simulink model "UNIFIER_dyn1"  (R2023b)
settings: Solver=VariableStepAuto  StartTime=0.0  StopTime=t_sim  RelTol=1e-3
InitFcn:
  | UNIFIER_LOAD
values from neighbouring files (symbols this model uses):
  b = 20.11467    [UNIFIER_LOAD.mat]
  c = 1.43676    [UNIFIER_LOAD.mat]
  dp_DEP =     [UNIFIER_LOAD.mat]
  dp_FUSE_FIN =     [UNIFIER_LOAD.mat]
  dp_HTU =     [UNIFIER_LOAD.mat]
  dp_VTAIL =     [UNIFIER_LOAD.mat]
  dp_VTAIL_INDUCED =     [UNIFIER_LOAD.mat]
  dp_WING_root =     [UNIFIER_LOAD.mat]
  dp_WING_tip =     [UNIFIER_LOAD.mat]
  I = [23600  0  -1740; 0  89800  0; -1740  0  102000]    [UNIFIER_LOAD.mat]
  m = 7057    [UNIFIER_LOAD.mat]
  rho0 = 1.11164259067    [UNIFIER_LOAD.mat]
  S = 29.98388    [UNIFIER_LOAD.mat]
  u0 = [0 0 0 0.436332312999 1 0 0]    [UNIFIER_LOAD.mat]    (also in UNIFIER_ROMdyn_w.m = X0(3); UNIFIER_dynamics.m = u; UNIFIER_dynamics0.m = u; UNIFIER_forces.m = u)
  Vrw0 = [18.7938524157 0 6.84040286651]    [UNIFIER_LOAD.mat]    (also in UNIFIER_dynamics.m = x(4:6); UNIFIER_dynamics0.m = x(4:6); UNIFIER_forces.m = x(4:6); UNIFIER_forces0.m = x(4:6))
  vtail_nodes = [-16.4894695282 -2.83441376686 -2.73765826225 -16.1370849609 -2.45649194717 -2.44886755943 -15.8320636749 -2.07857012749 -2.1468129158 -15.5873622894 -1.7006483078 -1.90353524685 ... (48 elements, 3x16)]    [UNIFIER_LOAD.mat]
  wing_nodes = [-7.70795631409 -9.67500019073 -0.98178178072 -7.66801691055 -8.6313495636 -1.01726543903 -7.65512371063 -7.83034992218 -1.03603482246 -7.6036362648 -6.84600019455 -1.09595656395 ... (42 elements, 3x14)]    [UNIFIER_LOAD.mat]
  x0 = [0 0 -1000 18.7938524157 0 6.84040286651 0 0.349065850399 0 0 0 0]    [UNIFIER_LOAD.mat]    (also in UNIFIER_ROMdyn_w.m = X0(1); UNIFIER_dynamics.m = x; UNIFIER_dynamics0.m = x; UNIFIER_forces.m = x)
  xyz_cg = [-8.09 0 -0.2]    [UNIFIER_LOAD.mat]
  xyz_DEP = [-6.9629998 -10.05 -0.90899998 -6.921 -8.4499998 -0.792 -6.8660002 -6.8499999 -0.82300001 -6.8099999 -5.25 -0.85000002 ... (36 elements, 3x12)]    [UNIFIER_LOAD.mat]
undefined symbols (not defined in the file or in its folder): OBM, unifier_obm
libraries: sharedutil x7, aerolibtransform2 x4, sharedtransform x2, matrix_library x1, shared6dofsys x1, shared6dof x1, simulink x1
(part 3 of 3)

== system UNIFIER_dyn1/UNIFIER OBM/Aero/WingForces/Right/WingRootForces/WingRootPreLookup ==
  flap_defl : Inport
  alpha : Inport  Port=2
  V_node : Inport  Port=3
  DEP_J : Inport  Port=4
  Constant8 : Constant  Value=0:4
  Prelookup : PreLookup  BreakpointsData=dp_WING_root.flap_defl  IndexSearchMethod=Linear search  BeginIndexSearchUsingPreviousIndexResult=on  UseLastBreakpoint=on
  Prelookup1 : PreLookup  BreakpointsData=dp_WING_root.alphas  IndexSearchMethod=Linear search  BeginIndexSearchUsingPreviousIndexResult=on  UseLastBreakpoint=on
  Prelookup2 : PreLookup  BreakpointsData=dp_WING_root.V  IndexSearchMethod=Linear search  BeginIndexSearchUsingPreviousIndexResult=on  UseLastBreakpoint=on
  Prelookup3 : PreLookup  BreakpointsData=dp_WING_root.DEP_J  IndexSearchMethod=Linear search  BeginIndexSearchUsingPreviousIndexResult=on  UseLastBreakpoint=on
  Out1 : Outport
  Out2 : Outport  Port=2
  Out3 : Outport  Port=3
  Out4 : Outport  Port=4
  Out6 : Outport  Port=5
  Out7 : Outport  Port=6
  Out8 : Outport  Port=7
  Out9 : Outport  Port=8
  Out5 : Outport  Port=9
  wires:
  Prelookup3/2 -> Out9/1
  Prelookup3/1 -> Out8/1
  Prelookup2/2 -> Out7/1
  Prelookup2/1 -> Out6/1
  DEP_J/1 -> Prelookup3/1
  V_node/1 -> Prelookup2/1
  flap_defl/1 -> Prelookup/1
  Prelookup1/1 -> Out3/1
  alpha/1 -> Prelookup1/1
  Prelookup/2 -> Out2/1
  Prelookup1/2 -> Out4/1
  Constant8/1 -> Out5/1
  Prelookup/1 -> Out1/1

== system UNIFIER_dyn1/UNIFIER OBM/Aero/WingForces/Right/WingTipForces/WingRootPreLookup ==
  ail_defl : Inport
  alpha : Inport  Port=2
  V_node : Inport  Port=3
  DEP_J : Inport  Port=4
  Constant8 : Constant  Value=0:1
  Prelookup : PreLookup  BreakpointsData=dp_WING_tip.ail_defl  IndexSearchMethod=Linear search  BeginIndexSearchUsingPreviousIndexResult=on  UseLastBreakpoint=on
  Prelookup1 : PreLookup  BreakpointsData=dp_WING_tip.alphas  IndexSearchMethod=Linear search  BeginIndexSearchUsingPreviousIndexResult=on  UseLastBreakpoint=on
  Prelookup2 : PreLookup  BreakpointsData=dp_WING_tip.V  IndexSearchMethod=Linear search  BeginIndexSearchUsingPreviousIndexResult=on  UseLastBreakpoint=on
  Prelookup3 : PreLookup  BreakpointsData=dp_WING_tip.DEP_J  IndexSearchMethod=Linear search  BeginIndexSearchUsingPreviousIndexResult=on  UseLastBreakpoint=on
  Out1 : Outport
  Out2 : Outport  Port=2
  Out3 : Outport  Port=3
  Out4 : Outport  Port=4
  Out6 : Outport  Port=5
  Out7 : Outport  Port=6
  Out8 : Outport  Port=7
  Out9 : Outport  Port=8
  Out5 : Outport  Port=9
  wires:
  Prelookup3/2 -> Out9/1
  Prelookup3/1 -> Out8/1
  Prelookup2/2 -> Out7/1
  Prelookup2/1 -> Out6/1
  DEP_J/1 -> Prelookup3/1
  V_node/1 -> Prelookup2/1
  ail_defl/1 -> Prelookup/1
  Prelookup1/1 -> Out3/1
  alpha/1 -> Prelookup1/1
  Prelookup/2 -> Out2/1
  Prelookup1/2 -> Out4/1
  Constant8/1 -> Out5/1
  Prelookup/1 -> Out1/1
